simulink model "colocviuFeedback"  (R2025b)
settings: Solver=VariableStepAuto  StartTime=0.0  StopTime=10.0  RelTol=1e-3

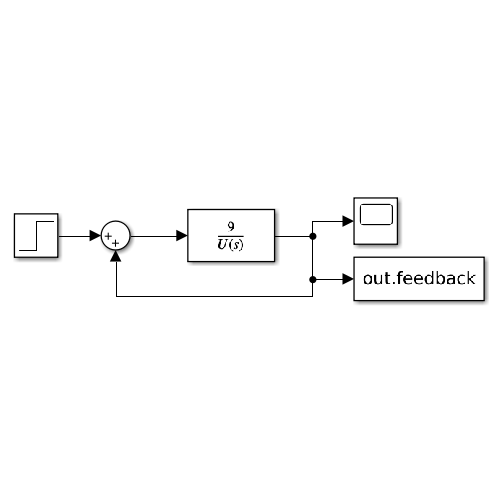
[thumbnail: Simulink's stored preview of the top-level diagram]
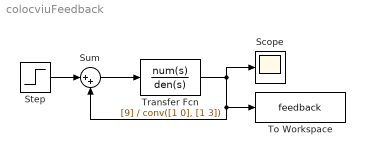
== system colocviuFeedback ==
  Scope : Scope
      settings: ActiveDisplayYMinimum=-1.5975543371411702E+6  ActiveDisplayYMaximum=1.4377989034270536E+7
  Step : Step  SampleTime=0
  Sum : Sum  Inputs=|++
  To Workspace : ToWorkspace  VariableName=feedback  SaveFormat=Timeseries  SampleTime=-1
  Transfer Fcn : TransferFcn  Numerator=[9]  Denominator=conv([1 0], [1 3])
  wires:
  Sum/1 -> Transfer Fcn/1
  Transfer Fcn/1 -> Scope/1, To Workspace/1, Sum/2
  Step/1 -> Sum/1
